simulink model "simulink_for_arduino_moore"  (R2019b)
settings: Solver=VariableStepAuto  StartTime=0.0  StopTime=inf  FixedStep=5000  RelTol=1e-3  EnableMultiTasking=on
libraries: arduinolib x9, simulink x6, dspswit3 x3
settings Model: SILPILModeSetting=veronly  ExtModeTrigDuration=2  Creator=Ahmed Zaghloul  LastModifiedBy=Bishoy Zaky
settings OptimizationCC: EnhancedBackFolding=on  PassReuseOutputArgsAs=Individual arguments  ZeroExternalMemoryAtStartup=off  ZeroInternalMemoryAtStartup=off  MaxStackSize=64  OptimizeBlockOrder=speed  DifferentSizesBufferReuse=on  OptimizationCustomize=off  EfficientTunableParamExpr=on
settings DebuggingCC: ParameterTunabilityLossMsg=error
settings HardwareCC: ProdBitPerInt=16  ProdBitPerPointer=16  ProdBitPerSizeT=16  ProdBitPerPtrDiffT=16  ProdLargestAtomicFloat=None  ProdWordSize=8  ProdHWDeviceType=Atmel->AVR
settings SFSimCC: MATLABDynamicMemAlloc=off
settings RTWCC: SystemTargetFile=ert.tlc  HardwareBoard=Arduino Uno  TLCOptions=-aInlineSetEventsForThisBaseRateFcn=TLC_FALSE -aSuppressMultiTaskScheduler=TLC_FALSE -aRateBasedStepFcn=1  TemplateMakefile=ert_default_tmf  Toolchain=Arduino AVR  BuildConfiguration=Faster Runs
settings CodeAppCC: ForceParamTrailComments=on  IgnoreCustomStorageClasses=off  OperatorAnnotations=on  SimulinkDataObjDesc=on  SFDataObjDesc=on  InsertBlockDesc=on
settings ERTTargetCC: SupportContinuousTime=on  SupportVariableSizeSignals=on  ExtModeStaticAllocSize=250

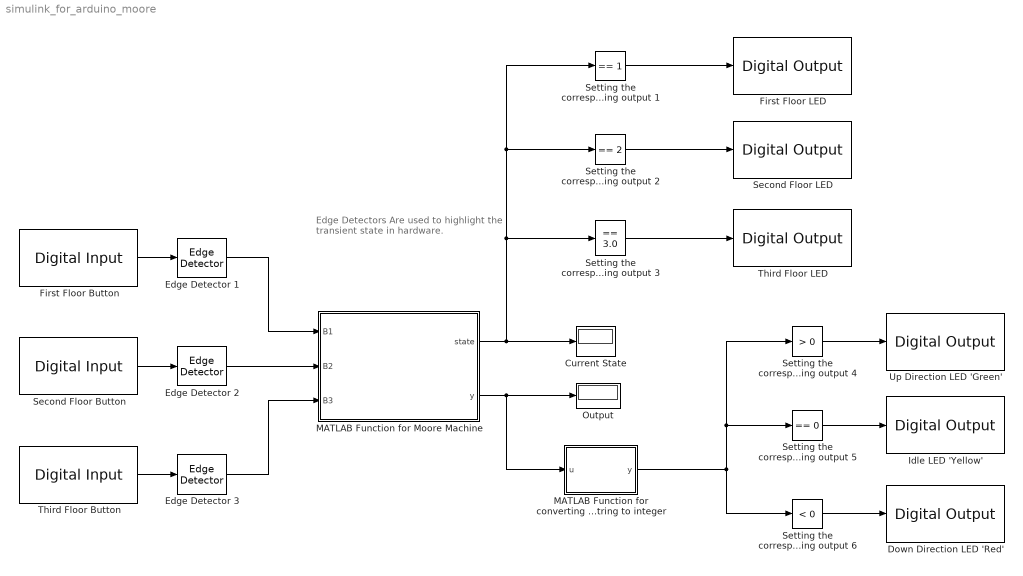
== system simulink_for_arduino_moore ==
  note: Edge Detectors Are used to highlight the transient state in hardware.
  Current State : Display
  Down Direction LED 'Red' : arduinolib/Digital Output  pinNumber=5  blockPlatform=arduino
  Edge Detector 1 : dspswit3/Edge Detector  InputProcessing=Columns as channels (frame based)
      settings: SourceProductBaseCode=DS
  Edge Detector 2 : dspswit3/Edge Detector  InputProcessing=Columns as channels (frame based)
      settings: SourceProductBaseCode=DS
  Edge Detector 3 : dspswit3/Edge Detector  InputProcessing=Columns as channels (frame based)
      settings: SourceProductBaseCode=DS
  First Floor Button : arduinolib/Digital Input  pinNumber=10  SampleTime=0.1  blockPlatform=arduino
  First Floor LED : arduinolib/Digital Output  pinNumber=2  blockPlatform=arduino
  Idle LED 'Yellow' : arduinolib/Digital Output  pinNumber=6  blockPlatform=arduino
  MATLAB Function for Moore Machine : MATLAB Function  TreatAsAtomicUnit=on
  MATLAB Function for converting output string to integer : MATLAB Function  TreatAsAtomicUnit=on
  "Output\t" : Display
  Second Floor Button : arduinolib/Digital Input  pinNumber=9  SampleTime=0.1  blockPlatform=arduino
  Second Floor LED : arduinolib/Digital Output  pinNumber=3  blockPlatform=arduino
  Setting the corresponding output 1 : simulink/Logic and Bit Operations/Compare To Constant  relop===  const=1  OutDataTypeStr=boolean
  Setting the corresponding output 2 : simulink/Logic and Bit Operations/Compare To Constant  relop===  const=2  OutDataTypeStr=boolean
  Setting the corresponding output 3 : simulink/Logic and Bit Operations/Compare To Constant  relop===  const=3.0  OutDataTypeStr=boolean
  Setting the corresponding output 4 : simulink/Logic and Bit Operations/Compare To Constant  relop=>  const=0  OutDataTypeStr=boolean
  Setting the corresponding output 5 : simulink/Logic and Bit Operations/Compare To Constant  relop===  const=0  OutDataTypeStr=boolean
  Setting the corresponding output 6 : simulink/Logic and Bit Operations/Compare To Constant  relop=<  const=0  OutDataTypeStr=boolean
  Third Floor Button : arduinolib/Digital Input  pinNumber=8  SampleTime=0.1  blockPlatform=arduino
  Third Floor LED : arduinolib/Digital Output  pinNumber=4  blockPlatform=arduino
  Up Direction LED 'Green' : arduinolib/Digital Output  pinNumber=7  blockPlatform=arduino
  wires:
  MATLAB Function for Moore Machine/1(state) -> Setting the corresponding output 1/1, Setting the corresponding output 2/1, Setting the corresponding output 3/1, Current State/1
  MATLAB Function for Moore Machine/2(y) -> "Output\t"/1, MATLAB Function for converting output string to integer/1(u)
  MATLAB Function for converting output string to integer/1(y) -> Setting the corresponding output 4/1, Setting the corresponding output 5/1, Setting the corresponding output 6/1
  Setting the corresponding output 1/1 -> First Floor LED/1
  Setting the corresponding output 2/1 -> Second Floor LED/1
  Setting the corresponding output 3/1 -> Third Floor LED/1
  Setting the corresponding output 6/1 -> Down Direction LED 'Red'/1
  Setting the corresponding output 5/1 -> Idle LED 'Yellow'/1
  Setting the corresponding output 4/1 -> Up Direction LED 'Green'/1
  First Floor Button/1 -> Edge Detector 1/1
  Second Floor Button/1 -> Edge Detector 2/1
  Third Floor Button/1 -> Edge Detector 3/1
  Edge Detector 1/1 -> MATLAB Function for Moore Machine/1(B1)
  Edge Detector 2/1 -> MATLAB Function for Moore Machine/2(B2)
  Edge Detector 3/1 -> MATLAB Function for Moore Machine/3(B3)

== matlab function simulink_for_arduino_moore/MATLAB Function for Moore Machine ==
  data: state output; B1 input; y output; B2 input; B3 input
function [state ,y] = fcn(B1,B2,B3)
persistent current_state
if(isempty(current_state))
    current_state = 1;
end
switch current_state
    case 1
        if(B1)
            current_state = 1;
        elseif(B2)
            current_state = 4;
        elseif(B3)
            current_state = 6;
        end
    case 2
        if(B1)
            current_state = 5;
        elseif(B2)
            current_state = 2;
        elseif(B3)
            current_state = 8;
        end
    case 3
        if(B1)
            current_state = 7;
        elseif(B2)
            current_state = 9;
        elseif(B3)
            current_state = 3;
        end
    case 4
        if(B2)
            current_state = 2;
        end
    case 5
        if(B1)
            current_state = 1;
        end
    case 6
        if(B3)
            current_state = 3;
        end  
    case 7
        if(B1)
            current_state = 1;
        end  
    case 8
        if(B3)
            current_state = 3;
        end  
    case 9
        if(B2)
            current_state = 2;
        end  
end
switch current_state
    case 1
        y = "s";
    case 2
        y = "s";
    case 3
        y = "s";
    case 4
        y = "u1";
    case 5
        y = "u1";
    case 6
        y = "u2";
    case 7
        y = "d2";
    case 8
        y = "u1";
    otherwise
        y = "d1";
end
state = current_state;
end

== matlab function simulink_for_arduino_moore/MATLAB Function for converting output string to integer ==
  data: u input; y output
function y = fcn(u)
if u == "s"
    y = 0;
elseif u == "u1"
    y = 1;
elseif u == "u2"
    y = 2;
elseif u == "d1"
    y = -1;
else
    y = -2;
end
